simulink model "martins_version"  (R2023b)
settings: Solver=VariableStepAuto  StartTime=0.0  StopTime=Tend  RelTol=1e-3
undefined symbols (not defined in the file): c_dc_si1, c_f, C_mv, dc_p_ref0, DiscIntNeverNeededParam, H_vsm, Ibase_hv, Ibase_lv, Ibase_mv, k_AD, k_d_vsm, k_decouple, k_ffv, k_ic, k_idc, k_mod, k_p_p_vsm, k_p_q_vsm, k_pc, k_pdc, KG_LL, KI_LL, ki_q, Kp_cc, KP_LL, kpu, kslope_VSC, l_f, l_f_si1, l_grid, L_mv, l_t_hvmv, l_t_mvlv, L_Virt, Lbase1v, len_hvac, omega_nom, phase_shift_test_state, phase_shifts, r_f, r_f_si1, r_grid, R_mv, r_t_hvmv, r_t_mvlv, R_Virt, rocof_slope, Rocof_test_state, Sbase1, Tchange_gfm_ref, Tdelay, Ti_cc, Tnu, Trocof_end, Trocof_start, Ts_power, v_dc_init, v_dc_ref0, Vbase_hv, Vbase_lv ... (+6)
libraries: slpidlib x6, spsFirstOrderFilterLib x3, cstblocks x1, simulink x1, spsSampleandHoldLib x1, spspowerguiLib x1
(part 2 of 3)

== system martins_version/GFC_WT/CurrentControl ==
  ref : Inport
  meas : Inport  Port=2
  V grid meas : Inport  Port=3
  Constant : Constant
  Demux : Demux  Outputs=[vect, vect]
  Demux1 : Demux  Outputs=[vect, vect]
  Demux2 : Demux  Outputs=[vect, vect]
  Gain1 : Gain  Gain=1/0.005
  Gain4 : Gain  Gain=l_f
  Gain5 : Gain  Gain=l_f
  Gain6 : Gain  Gain=1/0.005
  Integrator1 : Integrator
  Integrator3 : Integrator
  Mux : Mux  Inputs=[vect, vect]
  Mux1 : Mux  Inputs=3
  Mux2 : Mux  Inputs=3
  PID Controller : slpidlib/PID Controller  Controller=PI  Form=Ideal  TimeDomain=Continuous-time  UseExternalTs=off  SampleTime=-1  IntegratorMethod=Forward Euler  FilterMethod=Forward Euler  ControllerParametersSource=internal  P=Kp_cc  I=Ti_cc  UseKiTs=off  D=0  N=100  UseFilter=on  TunerSelectOption=Transfer Function Based (PID Tuner App)  InitialConditionSource=internal  InitialConditionForIntegrator=0  InitialConditionForFilter=0  DifferentiatorICPrevScaledInput=0  ExternalReset=none  TrackingMode=off  Kt=1  LimitOutput=off  SatLimitsSource=internal  UpperSaturationLimit=inf  LowerSaturationLimit=-inf  LinearizeAsGain=on  AntiWindupMode=none  Kb=1  LimitIntegrator=off  UpperIntegratorSaturationLimit=inf  LowerIntegratorSaturationLimit=-inf  POutMin=[]  POutMax=[]  IOutMin=[]  IOutMax=[]  DOutMin=[]  DOutMax=[]  NOutMin=[]  NOutMax=[]  SumOutMin=[]  SumOutMax=[]  SaturationOutMin=[]  SaturationOutMax=[]  PParamMin=[]  PParamMax=[]  IParamMin=[]  IParamMax=[]  DParamMin=[]  DParamMax=[]  NParamMin=[]  NParamMax=[]  KbParamMin=[]  KbParamMax=[]  KtParamMin=[]  KtParamMax=[]  KbOutMin=[]  KbOutMax=[]  KtOutMin=[]  KtOutMax=[]  IntegratorOutMin=[]  IntegratorOutMax=[]  FilterOutMin=[]  FilterOutMax=[]  SumI1OutMin=[]  SumI1OutMax=[]  SumI2OutMin=[]  SumI2OutMax=[]  SumI3OutMin=[]  SumI3OutMax=[]  SumI4OutMin=[]  SumI4OutMax=[]  SumDOutMin=[]  SumDOutMax=[]  DifferentiatorOutMin=[]  DifferentiatorOutMax=[]  FilterDiffOutCoefMin=[]  FilterDiffOutCoefMax=[]  ReciprocalOutMin=[]  ReciprocalOutMax=[]  SumDenOutMin=[]  SumDenOutMax=[]  SumNumOutMin=[]  SumNumOutMax=[]  DivideOutMin=[]  DivideOutMax=[]  UdiffTsProdOutMin=[]  UdiffTsProdOutMax=[]  NTsProdOutMin=[]  NTsProdOutMax=[]  UintegralTsProdOutMin=[]  UintegralTsProdOutMax=[]  UngainTsProdOutMin=[]  UngainTsProdOutMax=[]  ClampingZeroOutDataTypeStr=Inherit: Inherit via back propagation  ClampingZeroOutMin=[]  ClampingZeroOutMax=[]  FilterDenConstantOutDataTypeStr=Inherit: Inherit via back propagation  FilterDenConstantOutMin=[]  FilterDenConstantOutMax=[]  PCopyOutDataTypeStr=Inherit: Inherit via back propagation  PCopyOutMin=[]  PCopyOutMax=[]  NCopyOutDataTypeStr=Inherit: Inherit via back propagation  NCopyOutMin=[]  NCopyOutMax=[]  IntegratorContinuousStateAttributes=''  IntegratorStateMustResolveToSignalObject=off  IntegratorRTWStateStorageClass=Auto  FilterContinuousStateAttributes=''  FilterStateMustResolveToSignalObject=off  FilterRTWStateStorageClass=Auto  ParallelPVariant=Passthrough  IdealPVariant=InternalParameters  IVariant=InternalParameters  DVariant=Disabled  IntegratorVariant=Continuous  SatVariant=Disabled  AWVariant=Passthrough  PCopyVariant=Disabled  TRVariant=Disabled  FdbkBlocksVariant=Forward  IdealPFdbkVariant=Disabled  SatFdbkVariant=Disabled  DerivativeFilterVariant=Disabled  NVariant=Disabled  NCopyVariant=Disabled_SignalSpec  FilterICVariant=Disabled  IntegratorICVariant=InternalICs  ExternalResetVariant=Disabled  TRSumVariant=Passthrough  SumFdbkVariant=Disabled  SumVariant=Sum_PI  TsampFilterVariant=InternalTs  TsampNgainVariant=Passthrough  TsampIntegralVariant=Disabled_SignalSpec  ExternalSaturationOutDataTypeStr=Inherit: Same as second input
  PID Controller1 : slpidlib/PID Controller  Controller=PI  Form=Ideal  TimeDomain=Continuous-time  UseExternalTs=off  SampleTime=-1  IntegratorMethod=Forward Euler  FilterMethod=Forward Euler  ControllerParametersSource=internal  P=Kp_cc  I=1/Ti_cc  UseKiTs=off  D=0  N=100  UseFilter=on  TunerSelectOption=Transfer Function Based (PID Tuner App)  InitialConditionSource=internal  InitialConditionForIntegrator=1  InitialConditionForFilter=0  DifferentiatorICPrevScaledInput=0  ExternalReset=none  TrackingMode=off  Kt=1  LimitOutput=off  SatLimitsSource=internal  UpperSaturationLimit=inf  LowerSaturationLimit=-inf  LinearizeAsGain=on  AntiWindupMode=none  Kb=1  LimitIntegrator=off  UpperIntegratorSaturationLimit=inf  LowerIntegratorSaturationLimit=-inf  POutMin=[]  POutMax=[]  IOutMin=[]  IOutMax=[]  DOutMin=[]  DOutMax=[]  NOutMin=[]  NOutMax=[]  SumOutMin=[]  SumOutMax=[]  SaturationOutMin=[]  SaturationOutMax=[]  PParamMin=[]  PParamMax=[]  IParamMin=[]  IParamMax=[]  DParamMin=[]  DParamMax=[]  NParamMin=[]  NParamMax=[]  KbParamMin=[]  KbParamMax=[]  KtParamMin=[]  KtParamMax=[]  KbOutMin=[]  KbOutMax=[]  KtOutMin=[]  KtOutMax=[]  IntegratorOutMin=[]  IntegratorOutMax=[]  FilterOutMin=[]  FilterOutMax=[]  SumI1OutMin=[]  SumI1OutMax=[]  SumI2OutMin=[]  SumI2OutMax=[]  SumI3OutMin=[]  SumI3OutMax=[]  SumI4OutMin=[]  SumI4OutMax=[]  SumDOutMin=[]  SumDOutMax=[]  DifferentiatorOutMin=[]  DifferentiatorOutMax=[]  FilterDiffOutCoefMin=[]  FilterDiffOutCoefMax=[]  ReciprocalOutMin=[]  ReciprocalOutMax=[]  SumDenOutMin=[]  SumDenOutMax=[]  SumNumOutMin=[]  SumNumOutMax=[]  DivideOutMin=[]  DivideOutMax=[]  UdiffTsProdOutMin=[]  UdiffTsProdOutMax=[]  NTsProdOutMin=[]  NTsProdOutMax=[]  UintegralTsProdOutMin=[]  UintegralTsProdOutMax=[]  UngainTsProdOutMin=[]  UngainTsProdOutMax=[]  ClampingZeroOutDataTypeStr=Inherit: Inherit via back propagation  ClampingZeroOutMin=[]  ClampingZeroOutMax=[]  FilterDenConstantOutDataTypeStr=Inherit: Inherit via back propagation  FilterDenConstantOutMin=[]  FilterDenConstantOutMax=[]  PCopyOutDataTypeStr=Inherit: Inherit via back propagation  PCopyOutMin=[]  PCopyOutMax=[]  NCopyOutDataTypeStr=Inherit: Inherit via back propagation  NCopyOutMin=[]  NCopyOutMax=[]  IntegratorContinuousStateAttributes=''  IntegratorStateMustResolveToSignalObject=off  IntegratorRTWStateStorageClass=Auto  FilterContinuousStateAttributes=''  FilterStateMustResolveToSignalObject=off  FilterRTWStateStorageClass=Auto  ParallelPVariant=Passthrough  IdealPVariant=InternalParameters  IVariant=InternalParameters  DVariant=Disabled  IntegratorVariant=Continuous  SatVariant=Disabled  AWVariant=Passthrough  PCopyVariant=Disabled  TRVariant=Disabled  FdbkBlocksVariant=Forward  IdealPFdbkVariant=Disabled  SatFdbkVariant=Disabled  DerivativeFilterVariant=Disabled  NVariant=Disabled  NCopyVariant=Disabled_SignalSpec  FilterICVariant=Disabled  IntegratorICVariant=InternalICs  ExternalResetVariant=Disabled  TRSumVariant=Passthrough  SumFdbkVariant=Disabled  SumVariant=Sum_PI  TsampFilterVariant=InternalTs  TsampNgainVariant=Passthrough  TsampIntegralVariant=Disabled_SignalSpec  ExternalSaturationOutDataTypeStr=Inherit: Same as second input
  Sum1 : Sum  Inputs=|+-
  Sum2 : Sum  Inputs=+-|
  Sum3 : Sum  Inputs=|+-
  Sum4 : Sum  Inputs=++-
  Sum5 : Sum  Inputs=+++
  Sum6 : Sum  Inputs=|+-
  d-axis-control : Scope  NumInputPorts=3
  q-axis control : Scope  NumInputPorts=3
  Out1 : Outport
  wires:
  PID Controller1/1 -> Mux1/2, Sum4/2
  Mux2/1 -> q-axis control/2
  Mux1/1 -> d-axis-control/2
  Demux2/1 -> Sum6/1
  V grid meas/1 -> Demux2/1
  Sum5/1 -> Mux/2, q-axis control/3
  Demux2/2 -> Sum3/1
  Gain4/1 -> Sum5/1, Mux2/3
  Gain5/1 -> Sum4/3, Mux1/3
  Sum4/1 -> Mux/1, d-axis-control/3
  Sum2/1 -> q-axis control/1, PID Controller/1
  PID Controller/1 -> Sum5/2, Mux2/2
  Demux/1 -> Sum1/1
  Demux/2 -> Sum2/1
  Demux1/1 -> Sum1/2, Gain4/1
  Demux1/2 -> Gain5/1, Sum2/2
  meas/1 -> Demux1/1
  ref/1 -> Demux/1
  Sum1/1 -> PID Controller1/1, d-axis-control/1
  Mux/1 -> Out1/1
  Gain6/1 -> Integrator3/1
  Sum6/1 -> Gain6/1
  Integrator3/1 -> Sum4/1, Mux1/1, Sum6/2
  Gain1/1 -> Integrator1/1
  Sum3/1 -> Gain1/1
  Integrator1/1 -> Sum3/2, Sum5/3, Mux2/1

== system martins_version/GFC_WT/PLL>>grid1 ==
  note: inv ([  cos(wt)   sin(wt)
      |    -sin(wt)    cos(wt)   ])
  note: =
  note: [  al
      |     be  ]
  note: =
  note: [  al
      |     be  ]
  note: [ d
      |    q ]
  note: *
  note: [ d
      |    q ]
  note: [  cos(wt)   -sin(wt)
      |    sin(wt)    cos(wt)   ]
  note: *
  vgdq : Inport
  thetaPLL : Inport  Port=2
  Cos : Trigonometry  Operator=cos
  Demux1 : Demux  Outputs=2
  Display5 : Display
  Mux3 : Mux  Inputs=2
  Product{,1..3} (4 alike) : Product
  Sin : Trigonometry
  Sum : Sum  Inputs=+-
  Sum1 : Sum
  vgDQ : Outport  InitialOutput=[0,0]  VectorParamsAs1DForOutWhenUnconnected=off
  wires:
  vgdq/1 -> Demux1/1
  thetaPLL/1 -> Cos/1, Sin/1
  Sin/1 -> Product3/2, Product1/2
  Demux1/1 -> Product3/1, Product/1
  Cos/1 -> Product2/2, Product/2
  Product/1 -> Sum/1
  Demux1/2 -> Product2/1, Product1/1
  Product1/1 -> Sum/2
  Sum/1 -> Mux3/1
  Product2/1 -> Sum1/1
  Product3/1 -> Sum1/2
  Sum1/1 -> Mux3/2
  Mux3/1 -> Display5/1, vgDQ/1

== system martins_version/GFC_WT/PQ PCC ==
  note: PQ VSC bus
  IDQ : Inport
  VDQ : Inport  Port=2
  Demux7 : Demux  Outputs=[vect vect]
  Demux8 : Demux  Outputs=[vect vect]
  Product{1,3..5} (4 alike) : Product  InputSameDT=on  SaturateOnIntegerOverflow=on  OutDataTypeStr=Inherit: Same as first input
  Sum : Sum  InputSameDT=on  SaturateOnIntegerOverflow=on  OutDataTypeStr=Inherit: Same as first input
  Sum1 : Sum  Inputs=+-  InputSameDT=on  SaturateOnIntegerOverflow=on  OutDataTypeStr=Inherit: Same as first input
  P : Outport
  Q : Outport  Port=2
  wires:
  Product5/1 -> Sum1/2
  Product1/1 -> Sum1/1
  Demux8/2 -> Product1/1, Product4/1
  Demux7/1 -> Product1/2, Product3/1
  Demux8/1 -> Product5/1, Product3/2
  Product4/1 -> Sum/2
  Demux7/2 -> Product4/2, Product5/2
  Product3/1 -> Sum/1
  VDQ/1 -> Demux8/1
  Sum1/1 -> Q/1
  IDQ/1 -> Demux7/1
  Sum/1 -> P/1

== system martins_version/GFC_WT/PQ Virtual Bus1 ==
  note: PQ Virtual bus
  IDQ : Inport
  VDQ : Inport  Port=2
  Demux5 : Demux  Outputs=[vect vect]
  Demux6 : Demux  Outputs=[vect vect]
  Product{1,3..5} (4 alike) : Product  InputSameDT=on  SaturateOnIntegerOverflow=on  OutDataTypeStr=Inherit: Same as first input
  Sum : Sum  InputSameDT=on  SaturateOnIntegerOverflow=on  OutDataTypeStr=Inherit: Same as first input
  Sum1 : Sum  Inputs=+-  InputSameDT=on  SaturateOnIntegerOverflow=on  OutDataTypeStr=Inherit: Same as first input
  P : Outport
  Q : Outport  Port=2
  wires:
  Sum/1 -> P/1
  VDQ/1 -> Demux6/1
  IDQ/1 -> Demux5/1
  Sum1/1 -> Q/1
  Product5/1 -> Sum1/2
  Product1/1 -> Sum1/1
  Demux6/2 -> Product4/1, Product1/1
  Demux5/1 -> Product1/2, Product3/1
  Demux6/1 -> Product3/2, Product5/1
  Product4/1 -> Sum/2
  Demux5/2 -> Product5/2, Product4/2
  Product3/1 -> Sum/1

== system martins_version/GFC_WT/RL filter1 ==
  note: Inverter side inductor
  In1 : Inport
  In2 : Inport  Port=2
  In3 : Inport  Port=3
  In4 : Inport  Port=4
  In5 : Inport  Port=5
  1 : Gain  Gain=r_f*Zbase1v
  2 : Gain  Gain=1/(l_f*Lbase1v)
  3 : Gain  Gain=r_f*Zbase1v
  4 : Gain  Gain=1/(l_f*Lbase1v)
  Id : Scope
  Id_int : Integrator  UpperSaturationLimit=50  LowerSaturationLimit=-1000
  Iq : Scope
  Iq_int : Integrator  UpperSaturationLimit=50  LowerSaturationLimit=-1000
  L value : Constant  Value=l_f*Lbase1v  SampleTime=-1
  Product : Product
  Product1 : Product
  Product2 : Product
  Sum1 : Sum  Inputs=|+---
  Sum8 : Sum  Inputs=|+-+-
  id1 : Display
  Out1 : Outport
  Out2 : Outport  Port=2
  wires:
  In5/1 -> Product/1
  Product/1 -> [wL], id1/1
  L value/1 -> Product/2
  In1/1 -> Sum1/2
  In3/1 -> Sum1/1
  In4/1 -> Sum8/2
  In2/1 -> Sum8/1
  Product2/1 -> Sum8/3
  Iq_int/1 -> Iq/1, Product2/2, 3/1, Out1/1
  4/1 -> Iq_int/1
  Sum8/1 -> 2/1
  2/1 -> Id_int/1
  Sum1/1 -> 4/1
  3/1 -> Sum1/4
  Product1/1 -> Sum1/3
  1/1 -> Sum8/4
  Id_int/1 -> Product1/2, Out2/1, Id/1, 1/1
  [wL] -> Product1/1, Product2/1

== system martins_version/GFC_WT/Reactive Power //AVR ==
  note: Voltage control
  note: IQref
  Vmag : Inport
  Qmeas : Inport  Port=2
  Constant5 : Constant
  Gain1 : Gain  Gain=k_d_vsm
  Gain3 : Gain  Gain=1/ki_q
  Gain8 : Gain  Commented=through  Gain=1/Sbase1
  Gain9 : Gain  Gain=k_p_q_vsm
  I_Gain_I_d3 : Gain  Commented=on  Gain=kslope_VSC
  I_d_error{1,3..5} (4 alike) : Scope  Commented=on
  I_q_Ref1 : Constant  Commented=on  Value=ones(vect,1)  SampleTime=-1
  Integrator : Integrator  Commented=on  LimitOutput=on  UpperSaturationLimit=0.2  LowerSaturationLimit=-0.2
  Integrator1 : Integrator
  Kip1 : Gain  Commented=on  Gain=10
  Qmeas1 : InportShadow  Port=2
  Qref1 : Constant  Value=0.0
  Scope : Scope  NumInputPorts=4
  Scope7 : Scope  NumInputPorts=2
  Step : Step  Commented=on  Time=2  Before=1  SampleTime=0
  Step2 : Step  Commented=on  Time=2  After=0  SampleTime=0
  Sum1 : Sum  Commented=on  Inputs=|+-+
  Sum3 : Sum  Inputs=|-+
  Sum4 : Sum  Inputs=|++
  Sum7 : Sum  Inputs=|+-
  Transfer Fcn1 : TransferFcn  Numerator=[ki_q]  Denominator=[1 ki_q]
  V_nominal : Constant  Value=ones(vect,1)
  Delta_V : Outport
  V_ref_d : Outport  Port=2
  wires:
  Kip1/1 -> Integrator/1
  Step/1 -> Sum1/1
  I_Gain_I_d3/1 -> Sum1/3, I_d_error5/1
  Qmeas/1 -> I_Gain_I_d3/1, I_d_error4/1
  Sum1/1 -> Kip1/1
  Integrator/1 -> I_d_error3/1, Delta_V/1
  Vmag/1 -> I_d_error1/1, Sum1/2
  [Q_grid] -> Gain8/1  "Gen Reactive Power"
  Qmeas1/1 -> [Q_grid]
  V_nominal/1 -> Sum4/2
  Gain8/1 -> Sum3/1
  Qref1/1 -> Sum3/2
  Sum4/1 -> V_ref_d/1, [V_ref_gfm], Scope7/1, Scope/4  "Vref"
  Sum3/1 -> Sum7/1, Scope7/2, Scope/1  "delta Q"
  Integrator1/1 -> Scope/2, Gain9/1, Gain1/1
  Gain9/1 -> Scope/3, Sum4/1
  Constant5/1 -> ?
  Gain3/1 -> Integrator1/1
  Sum7/1 -> Gain3/1
  Gain1/1 -> Sum7/2

== system martins_version/GFC_WT/Subsystem ==
  In1 : Inport
  In2 : Inport  Port=2
  omega_PLL : Inport  Port=3
  omega_ref : Inport  Port=4
  In4 : Inport  Port=5
  Constant : Constant  Commented=on  Value=Tdelay*w_s
  Current Control : Subsystem  Commented=on
  Current Limit Logic : Subsystem  Commented=through
  Demux4 : Demux  Commented=on  Outputs=2
  First-Order Filter : spsFirstOrderFilterLib/First-Order Filter  Commented=on  FilterType=Lowpass  Tc=0.02  Ts=0  Initialize=on  Vac_Init=[0, 0, 60]  Vdc_Init=0  PlotResponse=off  FreqRange="[0,  200,  1]"
  From1 : From  Commented=on  GotoTag=Idq
  From17 : From  Commented=on  GotoTag=vQ
  From18 : From  Commented=on  GotoTag=vD
  From2 : From  Commented=on  GotoTag=thetaPLL
  From4 : From  Commented=on  GotoTag=vdq
  From5 : From  Commented=on  GotoTag=Iodq
  Goto3 : Goto  Commented=on  GotoTag=IQ
  Goto4 : Goto  Commented=on  GotoTag=ID
  I_d_error4 : Scope  Commented=on
  Kip6 : Gain  Commented=on  Gain=Vbase_lv
  Kip9 : Gain  Commented=through  Gain=1/Vbase_lv_pk
  PLL>>grid2 : Subsystem  Commented=on  AncestorBlock=powerlib_meascontrol/Transformations/Alpha-Beta-Zero to dq0/Subsystem - pi//2 delay
  Product : Product  Commented=on  Inputs=**  InputSameDT=on  SaturateOnIntegerOverflow=on  OutDataTypeStr=Inherit: Same as first input
  RL filter : Subsystem  Commented=on
      settings: PortSchema="{\"entries\":[{\"content\":{\"sides\":[{\"content\":{\"connectorIds\":[\"In1\",\"In2\",\"In3\",\"In4\"]},\"type\":\"ConnectorPlacement.EquallySpacedRectSide\",\"uuid\":\"57ad71d1-5664-4b35-a20c-d71f7e1cdc47\"},{\"content\":{\"connectorIds\":[\"Out1\",\"Out2\"],\"side\":\"RIGHT\"},\"type\":\"ConnectorPlacement.EquallySpacedRectSide\",\"uuid\":\"8101605d-eedb-4c26-847d-0cc0ce629d60\"},{\"content\":{\"connectorIds\":[],\"side\":\"TOP\"},\"type\":\"ConnectorPlacement.EquallySpacedRectSide\",\"uuid\":\"2627b00b-24a5-469a-be2d-9c3c8a1d2080\"},{\"content\":{\"connectorIds\":[\"In5\"],\"side\":\"BOTTOM\"},\"type\":\"ConnectorPlacement.EquallySpacedRectSide\",\"uuid\":\"fe553db7-7727-4a02-b1e7-5aedfb7840ee\"}]},\"type\":\"ConnectorPlacement.EquallySpacedConnector\",\"uuid\":\"f40200c8-ad5b-428c-8a4e-7641595b86c4\"}],\"packageUris\":[\"http://schema.mathworks.com/mf0/Connector/19700101\"],\"version\":\"1.0\"}"
  Step : Step  Commented=on  Before=1  After=0  SampleTime=0
  Sum1 : Sum  Commented=on  Inputs=|+-
  Sum2 : Sum  Commented=on  Inputs=|+-
  Switch : Switch  Commented=on  Criteria=u2 > Threshold  SaturateOnIntegerOverflow=off  InputSameDT=off
  Transport Delay : TransportDelay  Commented=on  DelayTime=Tdelay/2
  Transport Delay1 : TransportDelay  Commented=on  DelayTime=Tdelay/2
  Vdc value for converter AC output of 1 pu for m=1 : Constant  Commented=on  Value=1/k_mod
  Virtual Admittance1 : Subsystem  Commented=on
  Vmd13 : Display  Commented=on
  wires:
  Demux4/2 -> Transport Delay1/1
  Transport Delay/1 -> RL filter/2(In2)
  RL filter/2(Out2) -> Goto4/1
  Demux4/1 -> Transport Delay/1
  RL filter/1(Out1) -> Goto3/1
  Vdc value for converter AC output of 1 pu for m=1/1 -> Product/2
  Step/1 -> Switch/2
  Current Limit Logic/1(I_ref_sat) -> Current Control/1(i_cv_ref), Vmd13/1
  From17/1 -> RL filter/1(In1)
  omega_ref/1 -> RL filter/5(In5)
  From1/1 -> Current Control/3(i_o)
  Transport Delay1/1 -> RL filter/3(In3)
  Sum2/1 -> Virtual Admittance1/1(delvdq)
  Kip6/1 -> PLL>>grid2/1(vgdq)
  From4/1 -> Current Control/2(v_o)
  From18/1 -> RL filter/4(In4)
  Sum1/1 -> PLL>>grid2/2(thetaPLL)
  First-Order Filter/1 -> Current Limit Logic/1(I_ref_unsat)
  From2/1 -> Sum1/1
  Virtual Admittance1/1(Idqref) -> First-Order Filter/1
  Constant/1 -> Sum1/2
  From5/1 -> Current Control/4(i_cv)
  Switch/1 -> Product/1
  PLL>>grid2/1(vgDQ) -> I_d_error4/1, Demux4/1
  In1/1 -> Sum2/1, Switch/1
  Current Control/1(v_ref_dq) -> Switch/3
  Product/1 -> Kip6/1
  omega_PLL/1 -> Virtual Admittance1/2(omega_PLL)
  In2/1 -> Sum2/2
  Kip9/1 -> ?
  In4/1 -> Kip9/1

== system martins_version/GFC_WT/VoltageControl ==
  ref : Inport
  meas : Inport  Port=2
  I filter meas : Inport  Port=3
  Demux1 : Demux  Outputs=[vect, vect]
  Demux2 : Demux  Outputs=[vect, vect]
  Demux3 : Demux  Outputs=[vect, vect]
  Gain4 : Gain  Gain=0.0757204
  Gain5 : Gain  Gain=0.0757204
  Gain6 : Gain  Gain=1/0.005
  Gain7 : Gain  Gain=1/0.005
  Integrator3 : Integrator
  Integrator4 : Integrator
  Mux : Mux  Inputs=[vect, vect]
  Mux1 : Mux  Inputs=3
  Mux2 : Mux  Inputs=3
  PID Controller : slpidlib/PID Controller  Controller=PI  Form=Ideal  TimeDomain=Continuous-time  UseExternalTs=off  SampleTime=-1  IntegratorMethod=Forward Euler  FilterMethod=Forward Euler  ControllerParametersSource=internal  P=kpu  I=1/Tnu  UseKiTs=off  D=0  N=100  UseFilter=on  TunerSelectOption=Transfer Function Based (PID Tuner App)  InitialConditionSource=internal  InitialConditionForIntegrator=0  InitialConditionForFilter=0  DifferentiatorICPrevScaledInput=0  ExternalReset=none  TrackingMode=off  Kt=1  LimitOutput=off  SatLimitsSource=internal  UpperSaturationLimit=2  LowerSaturationLimit=-2  LinearizeAsGain=off  AntiWindupMode=none  Kb=1  LimitIntegrator=off  UpperIntegratorSaturationLimit=inf  LowerIntegratorSaturationLimit=-inf  POutMin=[]  POutMax=[]  IOutMin=[]  IOutMax=[]  DOutMin=[]  DOutMax=[]  NOutMin=[]  NOutMax=[]  SumOutMin=[]  SumOutMax=[]  SaturationOutMin=[]  SaturationOutMax=[]  PParamMin=[]  PParamMax=[]  IParamMin=[]  IParamMax=[]  DParamMin=[]  DParamMax=[]  NParamMin=[]  NParamMax=[]  KbParamMin=[]  KbParamMax=[]  KtParamMin=[]  KtParamMax=[]  KbOutMin=[]  KbOutMax=[]  KtOutMin=[]  KtOutMax=[]  IntegratorOutMin=[]  IntegratorOutMax=[]  FilterOutMin=[]  FilterOutMax=[]  SumI1OutMin=[]  SumI1OutMax=[]  SumI2OutMin=[]  SumI2OutMax=[]  SumI3OutMin=[]  SumI3OutMax=[]  SumI4OutMin=[]  SumI4OutMax=[]  SumDOutMin=[]  SumDOutMax=[]  DifferentiatorOutMin=[]  DifferentiatorOutMax=[]  FilterDiffOutCoefMin=[]  FilterDiffOutCoefMax=[]  ReciprocalOutMin=[]  ReciprocalOutMax=[]  SumDenOutMin=[]  SumDenOutMax=[]  SumNumOutMin=[]  SumNumOutMax=[]  DivideOutMin=[]  DivideOutMax=[]  UdiffTsProdOutMin=[]  UdiffTsProdOutMax=[]  NTsProdOutMin=[]  NTsProdOutMax=[]  UintegralTsProdOutMin=[]  UintegralTsProdOutMax=[]  UngainTsProdOutMin=[]  UngainTsProdOutMax=[]  ClampingZeroOutDataTypeStr=Inherit: Inherit via back propagation  ClampingZeroOutMin=[]  ClampingZeroOutMax=[]  FilterDenConstantOutDataTypeStr=Inherit: Inherit via back propagation  FilterDenConstantOutMin=[]  FilterDenConstantOutMax=[]  PCopyOutDataTypeStr=Inherit: Inherit via back propagation  PCopyOutMin=[]  PCopyOutMax=[]  NCopyOutDataTypeStr=Inherit: Inherit via back propagation  NCopyOutMin=[]  NCopyOutMax=[]  IntegratorContinuousStateAttributes=''  IntegratorStateMustResolveToSignalObject=off  IntegratorRTWStateStorageClass=Auto  FilterContinuousStateAttributes=''  FilterStateMustResolveToSignalObject=off  FilterRTWStateStorageClass=Auto  ParallelPVariant=Passthrough  IdealPVariant=InternalParameters  IVariant=InternalParameters  DVariant=Disabled  IntegratorVariant=Continuous  SatVariant=Disabled  AWVariant=Passthrough  PCopyVariant=Disabled  TRVariant=Disabled  FdbkBlocksVariant=Forward  IdealPFdbkVariant=Disabled  SatFdbkVariant=Disabled  DerivativeFilterVariant=Disabled  NVariant=Disabled  NCopyVariant=Disabled_SignalSpec  FilterICVariant=Disabled  IntegratorICVariant=InternalICs  ExternalResetVariant=Disabled  TRSumVariant=Passthrough  SumFdbkVariant=Disabled  SumVariant=Sum_PI  TsampFilterVariant=InternalTs  TsampNgainVariant=Passthrough  TsampIntegralVariant=Disabled_SignalSpec  ExternalSaturationOutDataTypeStr=Inherit: Same as second input
  PID Controller1 : slpidlib/PID Controller  Controller=PI  Form=Ideal  TimeDomain=Continuous-time  UseExternalTs=off  SampleTime=-1  IntegratorMethod=Forward Euler  FilterMethod=Forward Euler  ControllerParametersSource=internal  P=kpu  I=1/Tnu  UseKiTs=off  D=0  N=100  UseFilter=on  TunerSelectOption=Transfer Function Based (PID Tuner App)  InitialConditionSource=internal  InitialConditionForIntegrator=1  InitialConditionForFilter=0  DifferentiatorICPrevScaledInput=0  ExternalReset=none  TrackingMode=off  Kt=1  LimitOutput=off  SatLimitsSource=internal  UpperSaturationLimit=2  LowerSaturationLimit=-2  LinearizeAsGain=off  AntiWindupMode=none  Kb=1  LimitIntegrator=off  UpperIntegratorSaturationLimit=inf  LowerIntegratorSaturationLimit=-inf  POutMin=[]  POutMax=[]  IOutMin=[]  IOutMax=[]  DOutMin=[]  DOutMax=[]  NOutMin=[]  NOutMax=[]  SumOutMin=[]  SumOutMax=[]  SaturationOutMin=[]  SaturationOutMax=[]  PParamMin=[]  PParamMax=[]  IParamMin=[]  IParamMax=[]  DParamMin=[]  DParamMax=[]  NParamMin=[]  NParamMax=[]  KbParamMin=[]  KbParamMax=[]  KtParamMin=[]  KtParamMax=[]  KbOutMin=[]  KbOutMax=[]  KtOutMin=[]  KtOutMax=[]  IntegratorOutMin=[]  IntegratorOutMax=[]  FilterOutMin=[]  FilterOutMax=[]  SumI1OutMin=[]  SumI1OutMax=[]  SumI2OutMin=[]  SumI2OutMax=[]  SumI3OutMin=[]  SumI3OutMax=[]  SumI4OutMin=[]  SumI4OutMax=[]  SumDOutMin=[]  SumDOutMax=[]  DifferentiatorOutMin=[]  DifferentiatorOutMax=[]  FilterDiffOutCoefMin=[]  FilterDiffOutCoefMax=[]  ReciprocalOutMin=[]  ReciprocalOutMax=[]  SumDenOutMin=[]  SumDenOutMax=[]  SumNumOutMin=[]  SumNumOutMax=[]  DivideOutMin=[]  DivideOutMax=[]  UdiffTsProdOutMin=[]  UdiffTsProdOutMax=[]  NTsProdOutMin=[]  NTsProdOutMax=[]  UintegralTsProdOutMin=[]  UintegralTsProdOutMax=[]  UngainTsProdOutMin=[]  UngainTsProdOutMax=[]  ClampingZeroOutDataTypeStr=Inherit: Inherit via back propagation  ClampingZeroOutMin=[]  ClampingZeroOutMax=[]  FilterDenConstantOutDataTypeStr=Inherit: Inherit via back propagation  FilterDenConstantOutMin=[]  FilterDenConstantOutMax=[]  PCopyOutDataTypeStr=Inherit: Inherit via back propagation  PCopyOutMin=[]  PCopyOutMax=[]  NCopyOutDataTypeStr=Inherit: Inherit via back propagation  NCopyOutMin=[]  NCopyOutMax=[]  IntegratorContinuousStateAttributes=''  IntegratorStateMustResolveToSignalObject=off  IntegratorRTWStateStorageClass=Auto  FilterContinuousStateAttributes=''  FilterStateMustResolveToSignalObject=off  FilterRTWStateStorageClass=Auto  ParallelPVariant=Passthrough  IdealPVariant=InternalParameters  IVariant=InternalParameters  DVariant=Disabled  IntegratorVariant=Continuous  SatVariant=Disabled  AWVariant=Passthrough  PCopyVariant=Disabled  TRVariant=Disabled  FdbkBlocksVariant=Forward  IdealPFdbkVariant=Disabled  SatFdbkVariant=Disabled  DerivativeFilterVariant=Disabled  NVariant=Disabled  NCopyVariant=Disabled_SignalSpec  FilterICVariant=Disabled  IntegratorICVariant=InternalICs  ExternalResetVariant=Disabled  TRSumVariant=Passthrough  SumFdbkVariant=Disabled  SumVariant=Sum_PI  TsampFilterVariant=InternalTs  TsampNgainVariant=Passthrough  TsampIntegralVariant=Disabled_SignalSpec  ExternalSaturationOutDataTypeStr=Inherit: Same as second input
  Sum1 : Sum  Inputs=|+-
  Sum2 : Sum  Inputs=+-|
  Sum4 : Sum  Inputs=++-
  Sum5 : Sum  Inputs=+++
  Sum6 : Sum  Inputs=|+-
  Sum7 : Sum  Inputs=|+-
  d-axis v control : Scope  NumInputPorts=3
  q-axis v control : Scope  NumInputPorts=3
  i_dq_ref : Outport
  wires:
  Demux2/1 -> Sum6/1
  I filter meas/1 -> Demux2/1
  Sum5/1 -> Mux/2, q-axis v control/3
  Demux2/2 -> Sum7/1
  Sum4/1 -> Mux/1, d-axis v control/3
  Sum2/1 -> PID Controller/1, q-axis v control/1
  PID Controller/1 -> Mux1/2, Sum5/2
  ref/1 -> Demux3/1
  Demux3/2 -> Sum2/1
  Demux1/2 -> Gain4/1, Sum2/2
  meas/1 -> Demux1/1
  Sum1/1 -> PID Controller1/1, d-axis v control/1
  Mux/1 -> i_dq_ref/1
  Gain4/1 -> Mux2/3, Sum4/3
  Gain5/1 -> Mux1/3, Sum5/1
  Demux1/1 -> Sum1/2, Gain5/1
  PID Controller1/1 -> Mux2/2, Sum4/2
  Integrator3/1 -> Mux2/1, Sum4/1, Sum6/2
  Mux1/1 -> q-axis v control/2
  Mux2/1 -> d-axis v control/2
  Integrator4/1 -> Sum5/3, Mux1/1, Sum7/2
  Demux3/1 -> Sum1/1
  Gain6/1 -> Integrator3/1
  Sum6/1 -> Gain6/1
  Gain7/1 -> Integrator4/1
  Sum7/1 -> Gain7/1

== system martins_version/GFC_WT/grid>>PLL1 ==
  note: [  al
      |     be  ]
  note: [ d
      |    q ]
  note: [  cos(wt)   -sin(wt)
      |    sin(wt)    cos(wt)   ]
  note: =
  note: *
  note: [  al
      |     be  ]
  note: [ d
      |    q ]
  note: inv ([  cos(wt)   sin(wt)
      |    -sin(wt)    cos(wt)   ])
  note: =
  note: *
  vgDQ : Inport
  wt : Inport  Port=2
  Cos : Trigonometry  Operator=cos
  Demux1 : Demux  Outputs=[vect vect]
  Display5 : Display
  Mux3 : Mux  Inputs=2
  Product{,1..3} (4 alike) : Product
  Sin : Trigonometry
  Sum : Sum
  Sum1 : Sum  Inputs=+-
  vgdq : Outport  InitialOutput=[0,0]  VectorParamsAs1DForOutWhenUnconnected=off
  wires:
  Product3/1 -> Sum1/2
  Demux1/2 -> Product2/1, Product1/1
  Product2/1 -> Sum1/1
  Cos/1 -> Product2/2, Product/2
  Product1/1 -> Sum/2
  Sin/1 -> Product3/2, Product1/2
  vgDQ/1 -> Demux1/1
  Sum1/1 -> Mux3/2
  Mux3/1 -> vgdq/1, Display5/1
  Sum/1 -> Mux3/1
  Product/1 -> Sum/1
  wt/1 -> Cos/1, Sin/1
  Demux1/1 -> Product3/1, Product/1

== system martins_version/GFC_WT/grid>>PLL2 ==
  note: *
  note: =
  note: inv ([  cos(wt)   sin(wt)
      |    -sin(wt)    cos(wt)   ])
  note: [ d
      |    q ]
  note: [  al
      |     be  ]
  note: *
  note: =
  note: [  cos(wt)   -sin(wt)
      |    sin(wt)    cos(wt)   ]
  note: [ d
      |    q ]
  note: [  al
      |     be  ]
  vgDQ : Inport
  wt : Inport  Port=2
  Cos : Trigonometry  Operator=cos
  Demux1 : Demux  Outputs=2
  Display5 : Display
  Mux3 : Mux  Inputs=2
  Product{,1..3} (4 alike) : Product
  Sin : Trigonometry
  Sum : Sum
  Sum1 : Sum  Inputs=+-
  vgdq : Outport  InitialOutput=[0,0]  VectorParamsAs1DForOutWhenUnconnected=off
  wires:
  Demux1/1 -> Product/1, Product3/1
  wt/1 -> Sin/1, Cos/1
  Product/1 -> Sum/1
  Sum/1 -> Mux3/1
  Mux3/1 -> Display5/1, vgdq/1
  Sum1/1 -> Mux3/2
  vgDQ/1 -> Demux1/1
  Sin/1 -> Product1/2, Product3/2
  Product1/1 -> Sum/2
  Cos/1 -> Product/2, Product2/2
  Product2/1 -> Sum1/1
  Demux1/2 -> Product1/1, Product2/1
  Product3/1 -> Sum1/2

== system martins_version/GFC_WT/grid>>PLL3 ==
  note: *
  note: =
  note: inv ([  cos(wt)   sin(wt)
      |    -sin(wt)    cos(wt)   ])
  note: [ d
      |    q ]
  note: [  al
      |     be  ]
  note: *
  note: =
  note: [  cos(wt)   -sin(wt)
      |    sin(wt)    cos(wt)   ]
  note: [ d
      |    q ]
  note: [  al
      |     be  ]
  vgDQ : Inport
  wt : Inport  Port=2
  Cos : Trigonometry  Operator=cos
  Demux1 : Demux  Outputs=2
  Display5 : Display
  Mux3 : Mux  Inputs=[vect vect]
  Product{,1..3} (4 alike) : Product
  Sin : Trigonometry
  Sum : Sum
  Sum1 : Sum  Inputs=+-
  vgdq : Outport  InitialOutput=[0,0]  VectorParamsAs1DForOutWhenUnconnected=off
  wires:
  Demux1/1 -> Product/1, Product3/1
  wt/1 -> Sin/1, Cos/1
  Product/1 -> Sum/1
  Sum/1 -> Mux3/1
  Mux3/1 -> Display5/1, vgdq/1
  Sum1/1 -> Mux3/2
  vgDQ/1 -> Demux1/1
  Sin/1 -> Product1/2, Product3/2
  Product1/1 -> Sum/2
  Cos/1 -> Product/2, Product2/2
  Product2/1 -> Sum1/1
  Demux1/2 -> Product1/1, Product2/1
  Product3/1 -> Sum1/2

== system martins_version/GFC_WT/v_dc_reg ==
  In1 : Inport
  Ipart : DiscreteIntegrator  Commented=on  gainval=k_idc  SampleTime=-1  ICPrevOutput=DiscIntNeverNeededParam  ICPrevScaledInput=DiscIntNeverNeededParam
  PID Controller : slpidlib/PID Controller  Controller=PI  Form=Parallel  TimeDomain=Continuous-time  UseExternalTs=off  SampleTime=-1  IntegratorMethod=Forward Euler  FilterMethod=Forward Euler  ControllerParametersSource=internal  P=k_pdc  I=k_idc  UseKiTs=off  D=0  N=100  UseFilter=on  TunerSelectOption=Transfer Function Based (PID Tuner App)  InitialConditionSource=internal  InitialConditionForIntegrator=0  InitialConditionForFilter=0  DifferentiatorICPrevScaledInput=0  ExternalReset=none  TrackingMode=off  Kt=1  LimitOutput=off  SatLimitsSource=internal  UpperSaturationLimit=inf  LowerSaturationLimit=-inf  LinearizeAsGain=on  AntiWindupMode=none  Kb=1  LimitIntegrator=off  UpperIntegratorSaturationLimit=inf  LowerIntegratorSaturationLimit=-inf  POutMin=[]  POutMax=[]  IOutMin=[]  IOutMax=[]  DOutMin=[]  DOutMax=[]  NOutMin=[]  NOutMax=[]  SumOutMin=[]  SumOutMax=[]  SaturationOutMin=[]  SaturationOutMax=[]  PParamMin=[]  PParamMax=[]  IParamMin=[]  IParamMax=[]  DParamMin=[]  DParamMax=[]  NParamMin=[]  NParamMax=[]  KbParamMin=[]  KbParamMax=[]  KtParamMin=[]  KtParamMax=[]  KbOutMin=[]  KbOutMax=[]  KtOutMin=[]  KtOutMax=[]  IntegratorOutMin=[]  IntegratorOutMax=[]  FilterOutMin=[]  FilterOutMax=[]  SumI1OutMin=[]  SumI1OutMax=[]  SumI2OutMin=[]  SumI2OutMax=[]  SumI3OutMin=[]  SumI3OutMax=[]  SumI4OutMin=[]  SumI4OutMax=[]  SumDOutMin=[]  SumDOutMax=[]  DifferentiatorOutMin=[]  DifferentiatorOutMax=[]  FilterDiffOutCoefMin=[]  FilterDiffOutCoefMax=[]  ReciprocalOutMin=[]  ReciprocalOutMax=[]  SumDenOutMin=[]  SumDenOutMax=[]  SumNumOutMin=[]  SumNumOutMax=[]  DivideOutMin=[]  DivideOutMax=[]  UdiffTsProdOutMin=[]  UdiffTsProdOutMax=[]  NTsProdOutMin=[]  NTsProdOutMax=[]  UintegralTsProdOutMin=[]  UintegralTsProdOutMax=[]  UngainTsProdOutMin=[]  UngainTsProdOutMax=[]  ClampingZeroOutDataTypeStr=Inherit: Inherit via back propagation  ClampingZeroOutMin=[]  ClampingZeroOutMax=[]  FilterDenConstantOutDataTypeStr=Inherit: Inherit via back propagation  FilterDenConstantOutMin=[]  FilterDenConstantOutMax=[]  PCopyOutDataTypeStr=Inherit: Inherit via back propagation  PCopyOutMin=[]  PCopyOutMax=[]  NCopyOutDataTypeStr=Inherit: Inherit via back propagation  NCopyOutMin=[]  NCopyOutMax=[]  IntegratorContinuousStateAttributes=''  IntegratorStateMustResolveToSignalObject=off  IntegratorRTWStateStorageClass=Auto  FilterContinuousStateAttributes=''  FilterStateMustResolveToSignalObject=off  FilterRTWStateStorageClass=Auto  ParallelPVariant=InternalParameters  IdealPVariant=Disabled  IVariant=InternalParameters  DVariant=Disabled  IntegratorVariant=Continuous  SatVariant=Disabled  AWVariant=Passthrough  PCopyVariant=Disabled  TRVariant=Disabled  FdbkBlocksVariant=Forward  IdealPFdbkVariant=Disabled  SatFdbkVariant=Disabled  DerivativeFilterVariant=Disabled  NVariant=Disabled  NCopyVariant=Disabled_SignalSpec  FilterICVariant=Disabled  IntegratorICVariant=InternalICs  ExternalResetVariant=Disabled  TRSumVariant=Passthrough  SumFdbkVariant=Disabled  SumVariant=Sum_PI  TsampFilterVariant=InternalTs  TsampNgainVariant=Passthrough  TsampIntegralVariant=Disabled_SignalSpec  ExternalSaturationOutDataTypeStr=Inherit: Same as second input
  Ppart : Gain  Commented=on  Gain=k_pdc  SaturateOnIntegerOverflow=on  OutDataTypeStr=Inherit: Same as input  ParamDataTypeStr=Inherit: Same as input
  Sum5 : Sum  Commented=on  Inputs=|++  InputSameDT=on  SaturateOnIntegerOverflow=on  OutDataTypeStr=Inherit: Same as first input
  W : Outport
  wires:
  Ppart/1 -> Sum5/1
  Ipart/1 -> Sum5/2
  In1/1 -> PID Controller/1, Ppart/1, Ipart/1
  PID Controller/1 -> W/1

== system martins_version/HVAC CABLE 10 PI SEGMENTS 1/RC sys1 ==
  note: Left shunt capacitor
  note: shunt capacitor
  Iload_DQ : Inport
  "Isource_DQ " : Inport  Port=2
  omega_ref : Inport  Port=3
  1 : Gain  Gain=Rd
  10 : Gain  Gain=inv_Csource
  2 : Gain  Gain=Rd
  8 : Gain  Gain=Csource
  9 : Gain  Gain=inv_Csource
  Demux2 : Demux  Outputs=2
  Demux3 : Demux  Outputs=2
  Display1 : Display
  Display6 : Display
  Mux1 : Mux  Inputs=2
  Mux2 : Mux  Inputs=2
  Product7 : Product
  Product8 : Product
  Sum1 : Sum  Inputs=|++
  Sum14 : Sum  Inputs=|+--
  Sum15 : Sum  Inputs=|++-
  Sum2 : Sum  Inputs=|++
  Sum3 : Sum  Inputs=|+-
  Sum4 : Sum  Inputs=|+-
  Vcd : Scope
  VcpdR_int : Integrator  InitialCondition=VD0  UpperSaturationLimit=50  LowerSaturationLimit=-1000
  VcpqR_int : Integrator  InitialCondition=VQ0  UpperSaturationLimit=50  LowerSaturationLimit=-1000
  Vcq : Scope
  VpccR_DQ : Outport  VectorParamsAs1DForOutWhenUnconnected=off
  wires:
  8/1 -> [wcs], Display1/1
  Mux1/1 -> VpccR_DQ/1
  Product8/1 -> Sum14/3
  Sum15/1 -> 9/1
  10/1 -> VcpqR_int/1
  Product7/1 -> Sum15/1
  VcpqR_int/1 -> Mux2/1, Sum2/1, Product7/2, Vcq/1
  [wcs] -> Product7/1, Product8/1
  Sum14/1 -> 10/1
  9/1 -> VcpdR_int/1
  omega_ref/1 -> 8/1
  Demux2/1 -> Sum4/1, Sum15/2
  Demux2/2 -> Sum3/1, Sum14/1
  Iload_DQ/1 -> Demux2/1
  "Isource_DQ "/1 -> Demux3/1
  Demux3/2 -> Sum3/2, Sum14/2
  Demux3/1 -> Sum4/2, Sum15/3
  VcpdR_int/1 -> Mux2/2, Product8/2, Sum1/1
  Sum1/1 -> Mux1/1
  Sum2/1 -> Mux1/2
  1/1 -> Sum2/2
  2/1 -> Sum1/2
  Mux2/1 -> Display6/1
  Sum3/1 -> 1/1
  Sum4/1 -> 2/1

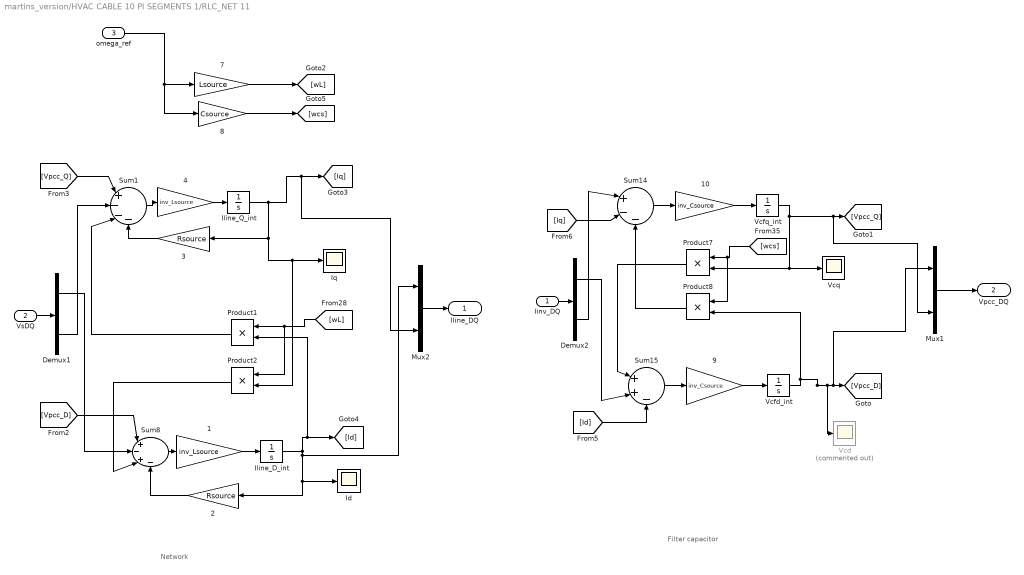
== system martins_version/HVAC CABLE 10 PI SEGMENTS 1/RLC_NET 11 ==
  note: Network
  note: Filter capacitor
  Iinv_DQ : Inport
  "VsDQ " : Inport  Port=2
  omega_ref : Inport  Port=3
  1 : Gain  Gain=inv_Lsource
  10 : Gain  Gain=inv_Csource
  2 : Gain  Gain=Rsource
  3 : Gain  Gain=Rsource
  4 : Gain  Gain=inv_Lsource
  7 : Gain  Gain=Lsource
  8 : Gain  Gain=Csource
  9 : Gain  Gain=inv_Csource
  Demux1 : Demux  Outputs=2
  Demux2 : Demux  Outputs=2
  Id : Scope
  Iline_D_int : Integrator  UpperSaturationLimit=50  LowerSaturationLimit=-1000
  Iline_Q_int : Integrator  UpperSaturationLimit=50  LowerSaturationLimit=-1000
  Iq : Scope
  Mux1 : Mux  Inputs=2
  Mux2 : Mux  Inputs=2
  Product{1..2,7..8} (4 alike) : Product
  Sum1 : Sum  Inputs=|+---
  Sum14 : Sum  Inputs=|+--
  Sum15 : Sum  Inputs=|++-
  Sum8 : Sum  Inputs=|+-+-
  Vcd : Scope  Commented=on
  Vcfd_int : Integrator  UpperSaturationLimit=50  LowerSaturationLimit=-1000
  Vcfq_int : Integrator  UpperSaturationLimit=50  LowerSaturationLimit=-1000
  Vcq : Scope
  Iline_DQ : Outport  VectorParamsAs1DForOutWhenUnconnected=off
  Vpcc_DQ : Outport  Port=2  VectorParamsAs1DForOutWhenUnconnected=off
  wires:
  Mux2/1 -> Iline_DQ/1
  Iinv_DQ/1 -> Demux2/1
  Demux2/2 -> Sum14/1
  Demux2/1 -> Sum15/2
  [wL] -> Product2/1, Product1/1
  Product1/1 -> Sum1/3
  4/1 -> Iline_Q_int/1
  3/1 -> Sum1/4
  Product2/1 -> Sum8/3
  2/1 -> Sum8/4
  Sum8/1 -> 1/1
  Iline_Q_int/1 -> 3/1, Product2/2, Iq/1, [Iq], Mux2/2
  Iline_D_int/1 -> Mux2/1, 2/1, Id/1, Product1/2, [Id]
  1/1 -> Iline_D_int/1
  Sum1/1 -> 4/1
  [Vpcc_D] -> Sum8/1
  [Vpcc_Q] -> Sum1/1
  omega_ref/1 -> 8/1, 7/1
  7/1 -> [wL]
  9/1 -> Vcfd_int/1
  Sum14/1 -> 10/1
  [wcs] -> Product8/1, Product7/1
  [Id] -> Sum15/3
  Vcfq_int/1 -> Mux1/2, [Vpcc_Q], Product7/2, Vcq/1
  Product7/1 -> Sum15/1
  [Iq] -> Sum14/2
  10/1 -> Vcfq_int/1
  Sum15/1 -> 9/1
  Product8/1 -> Sum14/3
  8/1 -> [wcs]
  Vcfd_int/1 -> Product8/2, Mux1/1, [Vpcc_D], Vcd/1
  Mux1/1 -> Vpcc_DQ/1
  Demux1/1 -> Sum8/2
  Demux1/2 -> Sum1/2
  "VsDQ "/1 -> Demux1/1

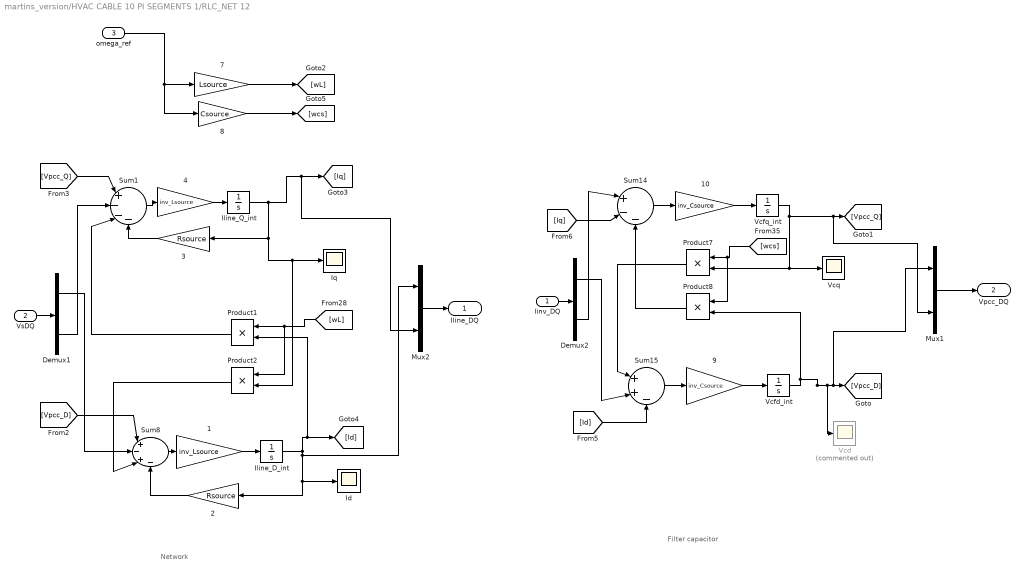
== system martins_version/HVAC CABLE 10 PI SEGMENTS 1/RLC_NET 12 ==
  note: Filter capacitor
  note: Network
  Iinv_DQ : Inport
  "VsDQ " : Inport  Port=2
  omega_ref : Inport  Port=3
  1 : Gain  Gain=inv_Lsource
  10 : Gain  Gain=inv_Csource
  2 : Gain  Gain=Rsource
  3 : Gain  Gain=Rsource
  4 : Gain  Gain=inv_Lsource
  7 : Gain  Gain=Lsource
  8 : Gain  Gain=Csource
  9 : Gain  Gain=inv_Csource
  Demux1 : Demux  Outputs=2
  Demux2 : Demux  Outputs=2
  Id : Scope
  Iline_D_int : Integrator  UpperSaturationLimit=50  LowerSaturationLimit=-1000
  Iline_Q_int : Integrator  UpperSaturationLimit=50  LowerSaturationLimit=-1000
  Iq : Scope
  Mux1 : Mux  Inputs=2
  Mux2 : Mux  Inputs=2
  Product{1..2,7..8} (4 alike) : Product
  Sum1 : Sum  Inputs=|+---
  Sum14 : Sum  Inputs=|+--
  Sum15 : Sum  Inputs=|++-
  Sum8 : Sum  Inputs=|+-+-
  Vcd : Scope  Commented=on
  Vcfd_int : Integrator  UpperSaturationLimit=50  LowerSaturationLimit=-1000
  Vcfq_int : Integrator  UpperSaturationLimit=50  LowerSaturationLimit=-1000
  Vcq : Scope
  Iline_DQ : Outport  VectorParamsAs1DForOutWhenUnconnected=off
  Vpcc_DQ : Outport  Port=2  VectorParamsAs1DForOutWhenUnconnected=off
  wires:
  "VsDQ "/1 -> Demux1/1
  Demux1/2 -> Sum1/2
  Demux1/1 -> Sum8/2
  Mux1/1 -> Vpcc_DQ/1
  Vcfd_int/1 -> Vcd/1, [Vpcc_D], Mux1/1, Product8/2
  8/1 -> [wcs]
  Product8/1 -> Sum14/3
  Sum15/1 -> 9/1
  10/1 -> Vcfq_int/1
  [Iq] -> Sum14/2
  Product7/1 -> Sum15/1
  Vcfq_int/1 -> Vcq/1, Product7/2, [Vpcc_Q], Mux1/2
  [Id] -> Sum15/3
  [wcs] -> Product7/1, Product8/1
  Sum14/1 -> 10/1
  9/1 -> Vcfd_int/1
  7/1 -> [wL]
  omega_ref/1 -> 7/1, 8/1
  [Vpcc_Q] -> Sum1/1
  [Vpcc_D] -> Sum8/1
  Sum1/1 -> 4/1
  1/1 -> Iline_D_int/1
  Iline_D_int/1 -> [Id], Product1/2, Id/1, 2/1, Mux2/1
  Iline_Q_int/1 -> Mux2/2, [Iq], Iq/1, Product2/2, 3/1
  Sum8/1 -> 1/1
  2/1 -> Sum8/4
  Product2/1 -> Sum8/3
  3/1 -> Sum1/4
  4/1 -> Iline_Q_int/1
  Product1/1 -> Sum1/3
  [wL] -> Product1/1, Product2/1
  Demux2/1 -> Sum15/2
  Demux2/2 -> Sum14/1
  Iinv_DQ/1 -> Demux2/1
  Mux2/1 -> Iline_DQ/1

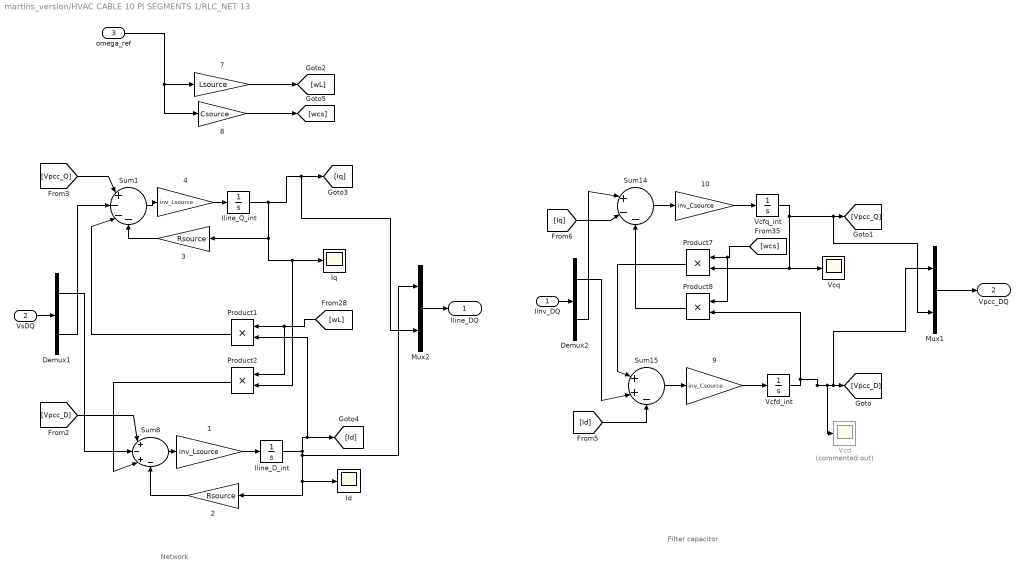
== system martins_version/HVAC CABLE 10 PI SEGMENTS 1/RLC_NET 13 ==
  note: Filter capacitor
  note: Network
  Iinv_DQ : Inport
  "VsDQ " : Inport  Port=2
  omega_ref : Inport  Port=3
  1 : Gain  Gain=inv_Lsource
  10 : Gain  Gain=inv_Csource
  2 : Gain  Gain=Rsource
  3 : Gain  Gain=Rsource
  4 : Gain  Gain=inv_Lsource
  7 : Gain  Gain=Lsource
  8 : Gain  Gain=Csource
  9 : Gain  Gain=inv_Csource
  Demux1 : Demux  Outputs=2
  Demux2 : Demux  Outputs=2
  Id : Scope
  Iline_D_int : Integrator  UpperSaturationLimit=50  LowerSaturationLimit=-1000
  Iline_Q_int : Integrator  UpperSaturationLimit=50  LowerSaturationLimit=-1000
  Iq : Scope
  Mux1 : Mux  Inputs=2
  Mux2 : Mux  Inputs=2
  Product{1..2,7..8} (4 alike) : Product
  Sum1 : Sum  Inputs=|+---
  Sum14 : Sum  Inputs=|+--
  Sum15 : Sum  Inputs=|++-
  Sum8 : Sum  Inputs=|+-+-
  Vcd : Scope  Commented=on
  Vcfd_int : Integrator  UpperSaturationLimit=50  LowerSaturationLimit=-1000
  Vcfq_int : Integrator  UpperSaturationLimit=50  LowerSaturationLimit=-1000
  Vcq : Scope
  Iline_DQ : Outport  VectorParamsAs1DForOutWhenUnconnected=off
  Vpcc_DQ : Outport  Port=2  VectorParamsAs1DForOutWhenUnconnected=off
  wires:
  "VsDQ "/1 -> Demux1/1
  Demux1/2 -> Sum1/2
  Demux1/1 -> Sum8/2
  Mux1/1 -> Vpcc_DQ/1
  Vcfd_int/1 -> Vcd/1, [Vpcc_D], Mux1/1, Product8/2
  8/1 -> [wcs]
  Product8/1 -> Sum14/3
  Sum15/1 -> 9/1
  10/1 -> Vcfq_int/1
  [Iq] -> Sum14/2
  Product7/1 -> Sum15/1
  Vcfq_int/1 -> Vcq/1, Product7/2, [Vpcc_Q], Mux1/2
  [Id] -> Sum15/3
  [wcs] -> Product7/1, Product8/1
  Sum14/1 -> 10/1
  9/1 -> Vcfd_int/1
  7/1 -> [wL]
  omega_ref/1 -> 7/1, 8/1
  [Vpcc_Q] -> Sum1/1
  [Vpcc_D] -> Sum8/1
  Sum1/1 -> 4/1
  1/1 -> Iline_D_int/1
  Iline_D_int/1 -> [Id], Product1/2, Id/1, 2/1, Mux2/1
  Iline_Q_int/1 -> Mux2/2, [Iq], Iq/1, Product2/2, 3/1
  Sum8/1 -> 1/1
  2/1 -> Sum8/4
  Product2/1 -> Sum8/3
  3/1 -> Sum1/4
  4/1 -> Iline_Q_int/1
  Product1/1 -> Sum1/3
  [wL] -> Product1/1, Product2/1
  Demux2/1 -> Sum15/2
  Demux2/2 -> Sum14/1
  Iinv_DQ/1 -> Demux2/1
  Mux2/1 -> Iline_DQ/1

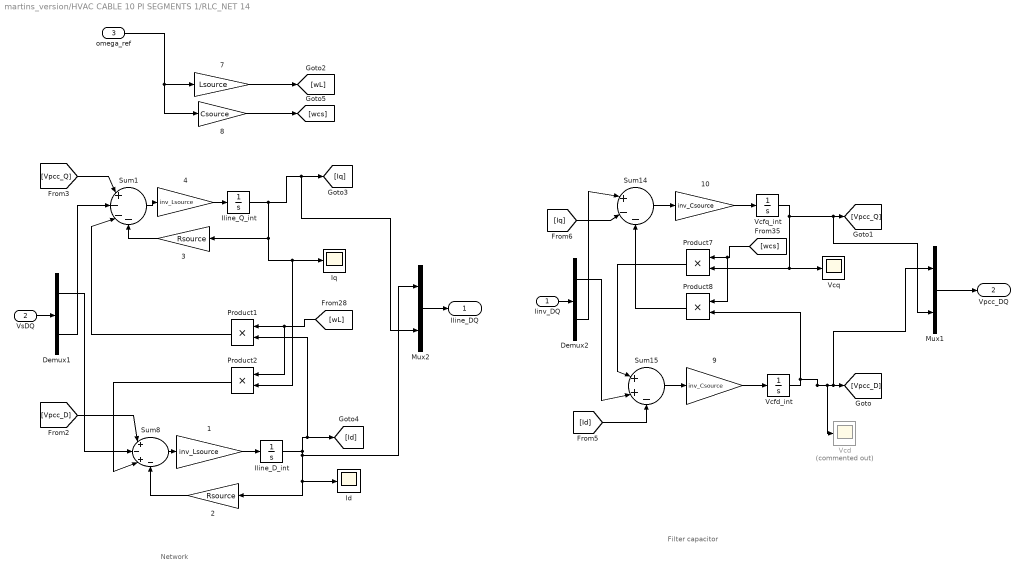
== system martins_version/HVAC CABLE 10 PI SEGMENTS 1/RLC_NET 14 ==
  note: Network
  note: Filter capacitor
  Iinv_DQ : Inport
  "VsDQ " : Inport  Port=2
  omega_ref : Inport  Port=3
  1 : Gain  Gain=inv_Lsource
  10 : Gain  Gain=inv_Csource
  2 : Gain  Gain=Rsource
  3 : Gain  Gain=Rsource
  4 : Gain  Gain=inv_Lsource
  7 : Gain  Gain=Lsource
  8 : Gain  Gain=Csource
  9 : Gain  Gain=inv_Csource
  Demux1 : Demux  Outputs=2
  Demux2 : Demux  Outputs=2
  Id : Scope
  Iline_D_int : Integrator  UpperSaturationLimit=50  LowerSaturationLimit=-1000
  Iline_Q_int : Integrator  UpperSaturationLimit=50  LowerSaturationLimit=-1000
  Iq : Scope
  Mux1 : Mux  Inputs=2
  Mux2 : Mux  Inputs=2
  Product{1..2,7..8} (4 alike) : Product
  Sum1 : Sum  Inputs=|+---
  Sum14 : Sum  Inputs=|+--
  Sum15 : Sum  Inputs=|++-
  Sum8 : Sum  Inputs=|+-+-
  Vcd : Scope  Commented=on
  Vcfd_int : Integrator  UpperSaturationLimit=50  LowerSaturationLimit=-1000
  Vcfq_int : Integrator  UpperSaturationLimit=50  LowerSaturationLimit=-1000
  Vcq : Scope
  Iline_DQ : Outport  VectorParamsAs1DForOutWhenUnconnected=off
  Vpcc_DQ : Outport  Port=2  VectorParamsAs1DForOutWhenUnconnected=off
  wires:
  Mux2/1 -> Iline_DQ/1
  Iinv_DQ/1 -> Demux2/1
  Demux2/2 -> Sum14/1
  Demux2/1 -> Sum15/2
  [wL] -> Product2/1, Product1/1
  Product1/1 -> Sum1/3
  4/1 -> Iline_Q_int/1
  3/1 -> Sum1/4
  Product2/1 -> Sum8/3
  2/1 -> Sum8/4
  Sum8/1 -> 1/1
  Iline_Q_int/1 -> 3/1, Product2/2, Iq/1, [Iq], Mux2/2
  Iline_D_int/1 -> Mux2/1, 2/1, Id/1, Product1/2, [Id]
  1/1 -> Iline_D_int/1
  Sum1/1 -> 4/1
  [Vpcc_D] -> Sum8/1
  [Vpcc_Q] -> Sum1/1
  omega_ref/1 -> 8/1, 7/1
  7/1 -> [wL]
  9/1 -> Vcfd_int/1
  Sum14/1 -> 10/1
  [wcs] -> Product8/1, Product7/1
  [Id] -> Sum15/3
  Vcfq_int/1 -> Mux1/2, [Vpcc_Q], Product7/2, Vcq/1
  Product7/1 -> Sum15/1
  [Iq] -> Sum14/2
  10/1 -> Vcfq_int/1
  Sum15/1 -> 9/1
  Product8/1 -> Sum14/3
  8/1 -> [wcs]
  Vcfd_int/1 -> Product8/2, Mux1/1, [Vpcc_D], Vcd/1
  Mux1/1 -> Vpcc_DQ/1
  Demux1/1 -> Sum8/2
  Demux1/2 -> Sum1/2
  "VsDQ "/1 -> Demux1/1

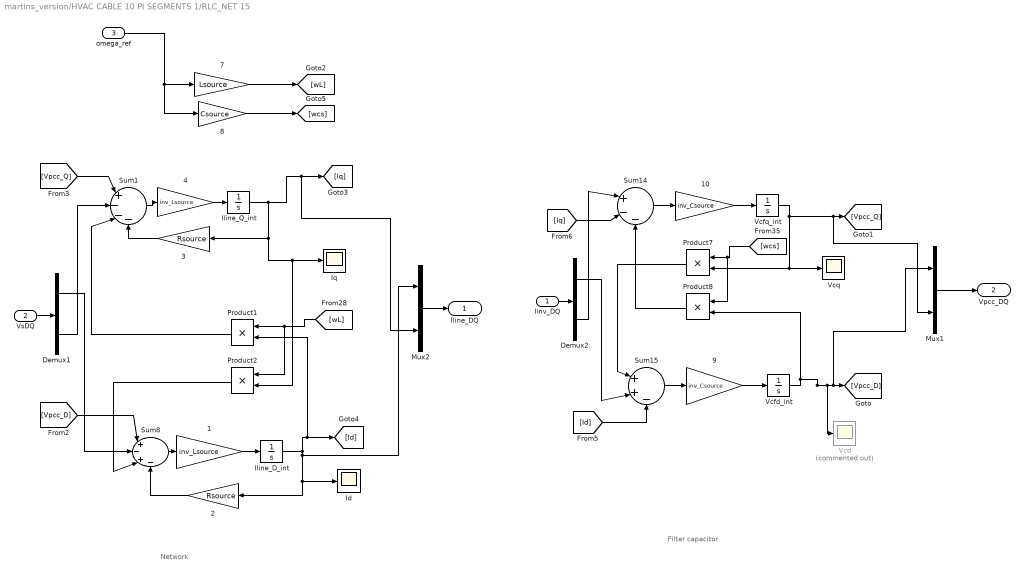
== system martins_version/HVAC CABLE 10 PI SEGMENTS 1/RLC_NET 15 ==
  note: Filter capacitor
  note: Network
  Iinv_DQ : Inport
  "VsDQ " : Inport  Port=2
  omega_ref : Inport  Port=3
  1 : Gain  Gain=inv_Lsource
  10 : Gain  Gain=inv_Csource
  2 : Gain  Gain=Rsource
  3 : Gain  Gain=Rsource
  4 : Gain  Gain=inv_Lsource
  7 : Gain  Gain=Lsource
  8 : Gain  Gain=Csource
  9 : Gain  Gain=inv_Csource
  Demux1 : Demux  Outputs=2
  Demux2 : Demux  Outputs=2
  Id : Scope
  Iline_D_int : Integrator  UpperSaturationLimit=50  LowerSaturationLimit=-1000
  Iline_Q_int : Integrator  UpperSaturationLimit=50  LowerSaturationLimit=-1000
  Iq : Scope
  Mux1 : Mux  Inputs=2
  Mux2 : Mux  Inputs=2
  Product{1..2,7..8} (4 alike) : Product
  Sum1 : Sum  Inputs=|+---
  Sum14 : Sum  Inputs=|+--
  Sum15 : Sum  Inputs=|++-
  Sum8 : Sum  Inputs=|+-+-
  Vcd : Scope  Commented=on
  Vcfd_int : Integrator  UpperSaturationLimit=50  LowerSaturationLimit=-1000
  Vcfq_int : Integrator  UpperSaturationLimit=50  LowerSaturationLimit=-1000
  Vcq : Scope
  Iline_DQ : Outport  VectorParamsAs1DForOutWhenUnconnected=off
  Vpcc_DQ : Outport  Port=2  VectorParamsAs1DForOutWhenUnconnected=off
  wires:
  "VsDQ "/1 -> Demux1/1
  Demux1/2 -> Sum1/2
  Demux1/1 -> Sum8/2
  Mux1/1 -> Vpcc_DQ/1
  Vcfd_int/1 -> Vcd/1, [Vpcc_D], Mux1/1, Product8/2
  8/1 -> [wcs]
  Product8/1 -> Sum14/3
  Sum15/1 -> 9/1
  10/1 -> Vcfq_int/1
  [Iq] -> Sum14/2
  Product7/1 -> Sum15/1
  Vcfq_int/1 -> Vcq/1, Product7/2, [Vpcc_Q], Mux1/2
  [Id] -> Sum15/3
  [wcs] -> Product7/1, Product8/1
  Sum14/1 -> 10/1
  9/1 -> Vcfd_int/1
  7/1 -> [wL]
  omega_ref/1 -> 7/1, 8/1
  [Vpcc_Q] -> Sum1/1
  [Vpcc_D] -> Sum8/1
  Sum1/1 -> 4/1
  1/1 -> Iline_D_int/1
  Iline_D_int/1 -> [Id], Product1/2, Id/1, 2/1, Mux2/1
  Iline_Q_int/1 -> Mux2/2, [Iq], Iq/1, Product2/2, 3/1
  Sum8/1 -> 1/1
  2/1 -> Sum8/4
  Product2/1 -> Sum8/3
  3/1 -> Sum1/4
  4/1 -> Iline_Q_int/1
  Product1/1 -> Sum1/3
  [wL] -> Product1/1, Product2/1
  Demux2/1 -> Sum15/2
  Demux2/2 -> Sum14/1
  Iinv_DQ/1 -> Demux2/1
  Mux2/1 -> Iline_DQ/1

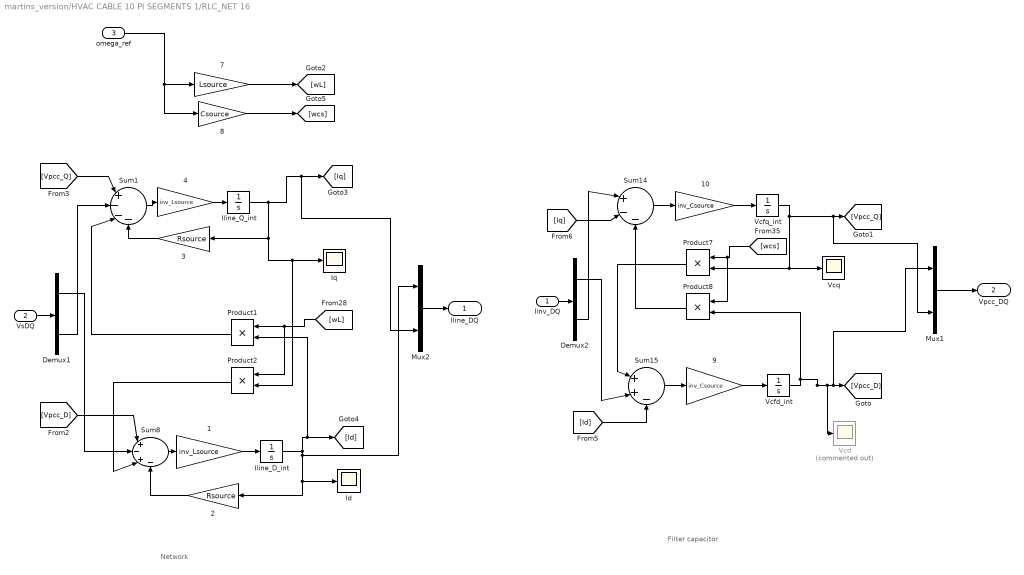
== system martins_version/HVAC CABLE 10 PI SEGMENTS 1/RLC_NET 16 ==
  note: Filter capacitor
  note: Network
  Iinv_DQ : Inport
  "VsDQ " : Inport  Port=2
  omega_ref : Inport  Port=3
  1 : Gain  Gain=inv_Lsource
  10 : Gain  Gain=inv_Csource
  2 : Gain  Gain=Rsource
  3 : Gain  Gain=Rsource
  4 : Gain  Gain=inv_Lsource
  7 : Gain  Gain=Lsource
  8 : Gain  Gain=Csource
  9 : Gain  Gain=inv_Csource
  Demux1 : Demux  Outputs=2
  Demux2 : Demux  Outputs=2
  Id : Scope
  Iline_D_int : Integrator  UpperSaturationLimit=50  LowerSaturationLimit=-1000
  Iline_Q_int : Integrator  UpperSaturationLimit=50  LowerSaturationLimit=-1000
  Iq : Scope
  Mux1 : Mux  Inputs=2
  Mux2 : Mux  Inputs=2
  Product{1..2,7..8} (4 alike) : Product
  Sum1 : Sum  Inputs=|+---
  Sum14 : Sum  Inputs=|+--
  Sum15 : Sum  Inputs=|++-
  Sum8 : Sum  Inputs=|+-+-
  Vcd : Scope  Commented=on
  Vcfd_int : Integrator  UpperSaturationLimit=50  LowerSaturationLimit=-1000
  Vcfq_int : Integrator  UpperSaturationLimit=50  LowerSaturationLimit=-1000
  Vcq : Scope
  Iline_DQ : Outport  VectorParamsAs1DForOutWhenUnconnected=off
  Vpcc_DQ : Outport  Port=2  VectorParamsAs1DForOutWhenUnconnected=off
  wires:
  "VsDQ "/1 -> Demux1/1
  Demux1/2 -> Sum1/2
  Demux1/1 -> Sum8/2
  Mux1/1 -> Vpcc_DQ/1
  Vcfd_int/1 -> Vcd/1, [Vpcc_D], Mux1/1, Product8/2
  8/1 -> [wcs]
  Product8/1 -> Sum14/3
  Sum15/1 -> 9/1
  10/1 -> Vcfq_int/1
  [Iq] -> Sum14/2
  Product7/1 -> Sum15/1
  Vcfq_int/1 -> Vcq/1, Product7/2, [Vpcc_Q], Mux1/2
  [Id] -> Sum15/3
  [wcs] -> Product7/1, Product8/1
  Sum14/1 -> 10/1
  9/1 -> Vcfd_int/1
  7/1 -> [wL]
  omega_ref/1 -> 7/1, 8/1
  [Vpcc_Q] -> Sum1/1
  [Vpcc_D] -> Sum8/1
  Sum1/1 -> 4/1
  1/1 -> Iline_D_int/1
  Iline_D_int/1 -> [Id], Product1/2, Id/1, 2/1, Mux2/1
  Iline_Q_int/1 -> Mux2/2, [Iq], Iq/1, Product2/2, 3/1
  Sum8/1 -> 1/1
  2/1 -> Sum8/4
  Product2/1 -> Sum8/3
  3/1 -> Sum1/4
  4/1 -> Iline_Q_int/1
  Product1/1 -> Sum1/3
  [wL] -> Product1/1, Product2/1
  Demux2/1 -> Sum15/2
  Demux2/2 -> Sum14/1
  Iinv_DQ/1 -> Demux2/1
  Mux2/1 -> Iline_DQ/1

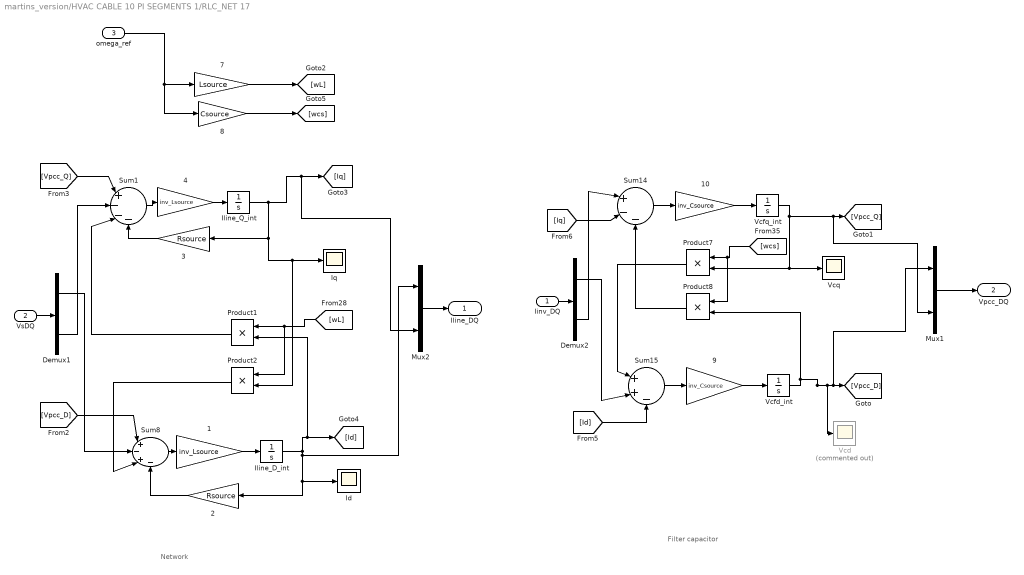
== system martins_version/HVAC CABLE 10 PI SEGMENTS 1/RLC_NET 17 ==
  note: Network
  note: Filter capacitor
  Iinv_DQ : Inport
  "VsDQ " : Inport  Port=2
  omega_ref : Inport  Port=3
  1 : Gain  Gain=inv_Lsource
  10 : Gain  Gain=inv_Csource
  2 : Gain  Gain=Rsource
  3 : Gain  Gain=Rsource
  4 : Gain  Gain=inv_Lsource
  7 : Gain  Gain=Lsource
  8 : Gain  Gain=Csource
  9 : Gain  Gain=inv_Csource
  Demux1 : Demux  Outputs=2
  Demux2 : Demux  Outputs=2
  Id : Scope
  Iline_D_int : Integrator  UpperSaturationLimit=50  LowerSaturationLimit=-1000
  Iline_Q_int : Integrator  UpperSaturationLimit=50  LowerSaturationLimit=-1000
  Iq : Scope
  Mux1 : Mux  Inputs=2
  Mux2 : Mux  Inputs=2
  Product{1..2,7..8} (4 alike) : Product
  Sum1 : Sum  Inputs=|+---
  Sum14 : Sum  Inputs=|+--
  Sum15 : Sum  Inputs=|++-
  Sum8 : Sum  Inputs=|+-+-
  Vcd : Scope  Commented=on
  Vcfd_int : Integrator  UpperSaturationLimit=50  LowerSaturationLimit=-1000
  Vcfq_int : Integrator  UpperSaturationLimit=50  LowerSaturationLimit=-1000
  Vcq : Scope
  Iline_DQ : Outport  VectorParamsAs1DForOutWhenUnconnected=off
  Vpcc_DQ : Outport  Port=2  VectorParamsAs1DForOutWhenUnconnected=off
  wires:
  Mux2/1 -> Iline_DQ/1
  Iinv_DQ/1 -> Demux2/1
  Demux2/2 -> Sum14/1
  Demux2/1 -> Sum15/2
  [wL] -> Product2/1, Product1/1
  Product1/1 -> Sum1/3
  4/1 -> Iline_Q_int/1
  3/1 -> Sum1/4
  Product2/1 -> Sum8/3
  2/1 -> Sum8/4
  Sum8/1 -> 1/1
  Iline_Q_int/1 -> 3/1, Product2/2, Iq/1, [Iq], Mux2/2
  Iline_D_int/1 -> Mux2/1, 2/1, Id/1, Product1/2, [Id]
  1/1 -> Iline_D_int/1
  Sum1/1 -> 4/1
  [Vpcc_D] -> Sum8/1
  [Vpcc_Q] -> Sum1/1
  omega_ref/1 -> 8/1, 7/1
  7/1 -> [wL]
  9/1 -> Vcfd_int/1
  Sum14/1 -> 10/1
  [wcs] -> Product8/1, Product7/1
  [Id] -> Sum15/3
  Vcfq_int/1 -> Mux1/2, [Vpcc_Q], Product7/2, Vcq/1
  Product7/1 -> Sum15/1
  [Iq] -> Sum14/2
  10/1 -> Vcfq_int/1
  Sum15/1 -> 9/1
  Product8/1 -> Sum14/3
  8/1 -> [wcs]
  Vcfd_int/1 -> Product8/2, Mux1/1, [Vpcc_D], Vcd/1
  Mux1/1 -> Vpcc_DQ/1
  Demux1/1 -> Sum8/2
  Demux1/2 -> Sum1/2
  "VsDQ "/1 -> Demux1/1
